simulink model "time_domain_exe1_autonomous"  (R2020b)
settings: Solver=VariableStepAuto  StartTime=0.0  StopTime=10.0  RelTol=1e-3
settings Model: Creator=petir  LastModifiedBy=petir

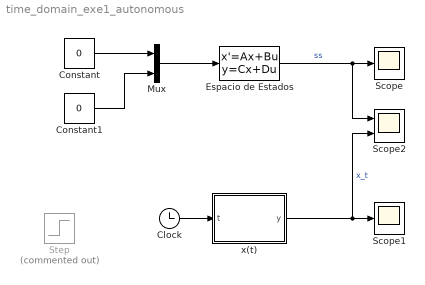
== system time_domain_exe1_autonomous ==
  Clock : Clock
  Constant : Constant  Value=0
  Constant1 : Constant  Value=0
  Espacio de Estados : StateSpace  A=[0, 1; -2 -3]  B=[0, 0; 0, 0]  C=[1, -1]  D=[0 0]  InitialCondition=[1; -1]
  Mux : Mux  Inputs=2
  Scope : Scope
  Scope1 : Scope
  Scope2 : Scope  NumInputPorts=2
  Step : Step  Commented=on  SampleTime=0
  x(t) : MATLAB Function  TreatAsAtomicUnit=on
  wires:
  Mux/1 -> Espacio de Estados/1
  Constant/1 -> Mux/1
  Constant1/1 -> Mux/2
  Espacio de Estados/1 -> Scope2/1, Scope/1  "ss"
  Clock/1 -> x(t)/1(t)
  x(t)/1(y) -> Scope2/2, Scope1/1  "x_t"

== matlab function time_domain_exe1_autonomous/x(t) ==
  data: t input; y output
function y = fcn(t)
x1 = exp(-t);
x2 = -exp(-t);
y = [x1; x2];
